simulink model "articulacion_q1"  (R2017b)
settings: Solver=VariableStepAuto  StartTime=0.0  StopTime=tmax  RelTol=1e-3
undefined symbols (not defined in the file): Beq, F_load_q1, f_pwm, Im_max, Jeq, Kdp, Kdv, Kip, Kiv, Km, Kpp, Kpv, Kt_q1, Kv_q1, Lm, Rm, ts, Vin_pwm, Vout_pwm
libraries: simulink x4
settings Model: Creator=JesusC  LastModifiedBy=JesusC

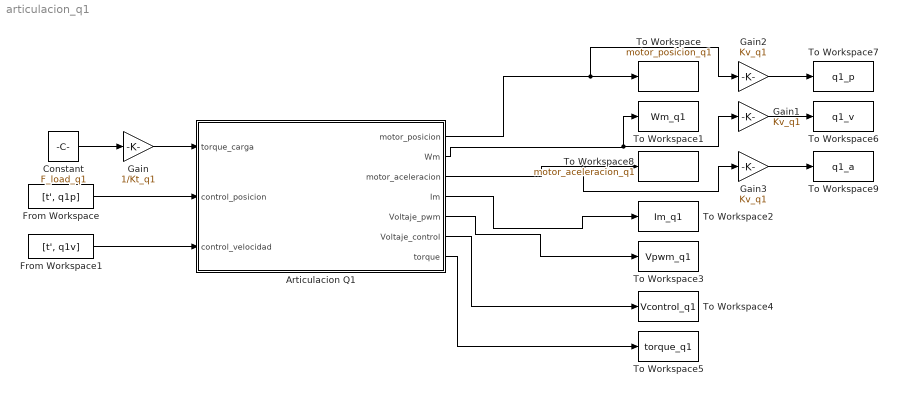
== system articulacion_q1 ==
  Articulacion Q1 : Subsystem
  Constant : Constant  Value=F_load_q1  VectorParams1D=off  SampleTime=ts
  From Workspace : FromWorkspace  VariableName=[t', q1p]  SampleTime=ts
  From Workspace1 : FromWorkspace  VariableName=[t', q1v]  SampleTime=ts
  Gain : Gain  Gain=1/Kt_q1
  Gain1 : Gain  Gain=Kv_q1
  Gain2 : Gain  Gain=Kv_q1
  Gain3 : Gain  Gain=Kv_q1
  To Workspace : ToWorkspace  VariableName=motor_posicion_q1  SampleTime=ts
      settings: MaxDataPoints=N
  To Workspace1 : ToWorkspace  VariableName=Wm_q1  SampleTime=ts
      settings: MaxDataPoints=N
  To Workspace2 : ToWorkspace  VariableName=Im_q1  SampleTime=ts
      settings: MaxDataPoints=N
  To Workspace3 : ToWorkspace  VariableName=Vpwm_q1  SampleTime=ts
      settings: MaxDataPoints=N
  To Workspace4 : ToWorkspace  VariableName=Vcontrol_q1  SampleTime=ts
      settings: MaxDataPoints=N
  To Workspace5 : ToWorkspace  VariableName=torque_q1  SampleTime=ts
      settings: MaxDataPoints=N
  To Workspace6 : ToWorkspace  VariableName=q1_v  SampleTime=ts
      settings: MaxDataPoints=N
  To Workspace7 : ToWorkspace  VariableName=q1_p  SampleTime=ts
      settings: MaxDataPoints=N
  To Workspace8 : ToWorkspace  VariableName=motor_aceleracion_q1  SampleTime=ts
      settings: MaxDataPoints=N
  To Workspace9 : ToWorkspace  VariableName=q1_a  SampleTime=ts
      settings: MaxDataPoints=N
  wires:
  Constant/1 -> Gain/1
  Gain1/1 -> To Workspace6/1
  Gain2/1 -> To Workspace7/1
  Articulacion Q1/6(Voltaje_control) -> To Workspace4/1
  Articulacion Q1/7(torque) -> To Workspace5/1
  Articulacion Q1/5(Voltaje_pwm) -> To Workspace3/1
  Articulacion Q1/4(Im) -> To Workspace2/1
  Articulacion Q1/2(Wm) -> Gain1/1, To Workspace1/1
  Articulacion Q1/1(motor_posicion) -> Gain2/1, To Workspace/1
  Articulacion Q1/3(motor_aceleracion) -> Gain3/1, To Workspace8/1
  Gain3/1 -> To Workspace9/1
  Gain/1 -> Articulacion Q1/1(torque_carga)
  From Workspace/1 -> Articulacion Q1/2(control_posicion)
  From Workspace1/1 -> Articulacion Q1/3(control_velocidad)

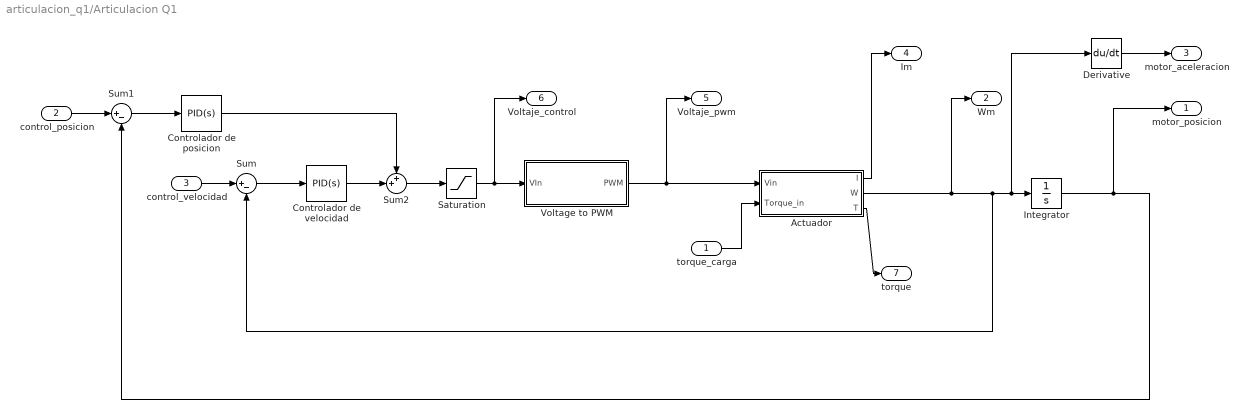
== system articulacion_q1/Articulacion Q1 ==
  torque_carga : Inport
  control_posicion : Inport  Port=2
  control_velocidad : Inport  Port=3
  "Actuador " : Subsystem
  Controlador de posicion : simulink/Continuous/PID Controller  Controller=PID  TimeDomain=Continuous-time  SampleTime=-1  IntegratorMethod=Forward Euler  FilterMethod=Forward Euler  Form=Parallel  UseFilter=on  ControllerParametersSource=internal  P=Kpp  I=Kip  D=Kdp  N=10000  InitialConditionSource=internal  InitialConditionForIntegrator=0  InitialConditionForFilter=0  ExternalReset=none  LimitOutput=off  UpperSaturationLimit=inf  LowerSaturationLimit=-inf  LinearizeAsGain=on  AntiWindupMode=none  Kb=1  TrackingMode=off  Kt=1  PParamMin=[]  PParamMax=[]  IParamMin=[]  IParamMax=[]  DParamMin=[]  DParamMax=[]  NParamMin=[]  NParamMax=[]  KbParamMin=[]  KbParamMax=[]  KtParamMin=[]  KtParamMax=[]  POutMin=[]  POutMax=[]  IOutMin=[]  IOutMax=[]  DOutMin=[]  DOutMax=[]  NOutMin=[]  NOutMax=[]  KbOutMin=[]  KbOutMax=[]  KtOutMin=[]  KtOutMax=[]  IntegratorOutMin=[]  IntegratorOutMax=[]  FilterOutMin=[]  FilterOutMax=[]  SumOutMin=[]  SumOutMax=[]  SumI1OutMin=[]  SumI1OutMax=[]  SumI2OutMin=[]  SumI2OutMax=[]  SumI3OutMin=[]  SumI3OutMax=[]  SumDOutMin=[]  SumDOutMax=[]  SaturationOutMin=[]  SaturationOutMax=[]  IntegratorContinuousStateAttributes=''  IntegratorStateMustResolveToSignalObject=off  IntegratorRTWStateStorageClass=Auto  FilterContinuousStateAttributes=''  FilterStateMustResolveToSignalObject=off  FilterRTWStateStorageClass=Auto  DifferentiatorICPrevScaledInput=0  DifferentiatorOutMin=[]  DifferentiatorOutMax=[]  InitialConditionSetting=State (most efficient)  FilterDiffOutCoefMin=[]  FilterDiffOutCoefMax=[]  SumDenOutMin=[]  SumDenOutMax=[]  SumNumOutMin=[]  SumNumOutMax=[]  ReciprocalOutMin=[]  ReciprocalOutMax=[]  DivideOutMin=[]  DivideOutMax=[]  TunerSelectOption=Transfer Function Based (PID Tuner App)
  Controlador de velocidad : simulink/Continuous/PID Controller  Controller=PID  TimeDomain=Continuous-time  SampleTime=-1  IntegratorMethod=Forward Euler  FilterMethod=Forward Euler  Form=Parallel  UseFilter=on  ControllerParametersSource=internal  P=Kpv  I=Kiv  D=Kdv  N=10000  InitialConditionSource=internal  InitialConditionForIntegrator=0  InitialConditionForFilter=0  ExternalReset=none  LimitOutput=off  UpperSaturationLimit=inf  LowerSaturationLimit=-inf  LinearizeAsGain=on  AntiWindupMode=none  Kb=1  TrackingMode=off  Kt=1  PParamMin=[]  PParamMax=[]  IParamMin=[]  IParamMax=[]  DParamMin=[]  DParamMax=[]  NParamMin=[]  NParamMax=[]  KbParamMin=[]  KbParamMax=[]  KtParamMin=[]  KtParamMax=[]  POutMin=[]  POutMax=[]  IOutMin=[]  IOutMax=[]  DOutMin=[]  DOutMax=[]  NOutMin=[]  NOutMax=[]  KbOutMin=[]  KbOutMax=[]  KtOutMin=[]  KtOutMax=[]  IntegratorOutMin=[]  IntegratorOutMax=[]  FilterOutMin=[]  FilterOutMax=[]  SumOutMin=[]  SumOutMax=[]  SumI1OutMin=[]  SumI1OutMax=[]  SumI2OutMin=[]  SumI2OutMax=[]  SumI3OutMin=[]  SumI3OutMax=[]  SumDOutMin=[]  SumDOutMax=[]  SaturationOutMin=[]  SaturationOutMax=[]  IntegratorContinuousStateAttributes=''  IntegratorStateMustResolveToSignalObject=off  IntegratorRTWStateStorageClass=Auto  FilterContinuousStateAttributes=''  FilterStateMustResolveToSignalObject=off  FilterRTWStateStorageClass=Auto  DifferentiatorICPrevScaledInput=0  DifferentiatorOutMin=[]  DifferentiatorOutMax=[]  InitialConditionSetting=State (most efficient)  FilterDiffOutCoefMin=[]  FilterDiffOutCoefMax=[]  SumDenOutMin=[]  SumDenOutMax=[]  SumNumOutMin=[]  SumNumOutMax=[]  ReciprocalOutMin=[]  ReciprocalOutMax=[]  DivideOutMin=[]  DivideOutMax=[]  TunerSelectOption=Transfer Function Based (PID Tuner App)
  Derivative : Derivative  CoefficientInTFapproximation=0
  Integrator : Integrator
  Saturation : Saturate  UpperLimit=Vin_pwm  LowerLimit=-Vin_pwm
  Sum : Sum  Inputs=|+-
  Sum1 : Sum  Inputs=|+-
  Sum2 : Sum  Inputs=++|
  Voltage to PWM : Subsystem
  motor_posicion : Outport
  Wm : Outport  Port=2
  motor_aceleracion : Outport  Port=3
  Im : Outport  Port=4
  Voltaje_pwm : Outport  Port=5
  Voltaje_control : Outport  Port=6
  torque : Outport  Port=7
  wires:
  Derivative/1 -> motor_aceleracion/1
  Integrator/1 -> motor_posicion/1, Sum1/2
  control_posicion/1 -> Sum1/1
  "Actuador "/1(I) -> Im/1
  "Actuador "/3(T) -> torque/1
  Sum2/1 -> Saturation/1
  Sum1/1 -> Controlador de posicion/1
  torque_carga/1 -> "Actuador "/2(Torque_in)
  Voltage to PWM/1(PWM) -> Voltaje_pwm/1, "Actuador "/1(Vin)
  Saturation/1 -> Voltaje_control/1, Voltage to PWM/1(VIn)
  control_velocidad/1 -> Sum/1
  "Actuador "/2(W) -> Wm/1, Sum/2, Derivative/1, Integrator/1
  Sum/1 -> Controlador de velocidad/1
  Controlador de velocidad/1 -> Sum2/2
  Controlador de posicion/1 -> Sum2/1

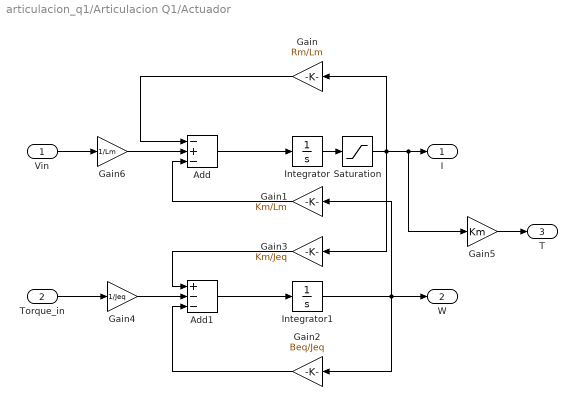
== system articulacion_q1/Articulacion Q1/Actuador  ==
  Vin : Inport
  Torque_in : Inport  Port=2
  Add : Sum  Inputs=-+-
  Add1 : Sum  Inputs=+--
  Gain : Gain  Gain=Rm/Lm
  Gain1 : Gain  Gain=Km/Lm
  Gain2 : Gain  Gain=Beq/Jeq
  Gain3 : Gain  Gain=Km/Jeq
  Gain4 : Gain  Gain=1/Jeq
  Gain5 : Gain  Gain=Km
  Gain6 : Gain  Gain=1/Lm
  Integrator : Integrator
  Integrator1 : Integrator
  Saturation : Saturate  UpperLimit=Im_max  LowerLimit=-Im_max
  I : Outport
  W : Outport  Port=2
  T : Outport  Port=3
  wires:
  Integrator/1 -> Saturation/1
  Gain/1 -> Add/1
  Integrator1/1 -> Gain2/1, Gain1/1, W/1
  Gain1/1 -> Add/3
  Add/1 -> Integrator/1
  Add1/1 -> Integrator1/1
  Gain2/1 -> Add1/3
  Gain3/1 -> Add1/1
  Torque_in/1 -> Gain4/1
  Gain4/1 -> Add1/2
  Gain5/1 -> T/1
  Vin/1 -> Gain6/1
  Gain6/1 -> Add/2
  Saturation/1 -> Gain3/1, Gain/1, Gain5/1, I/1

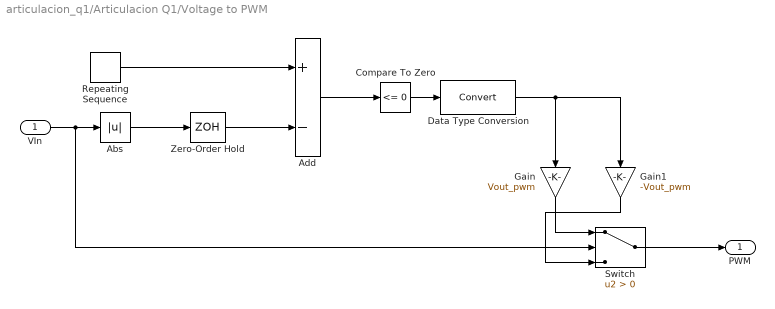
== system articulacion_q1/Articulacion Q1/Voltage to PWM ==
  VIn : Inport
  Abs : Abs
  Add : Sum  Inputs=+-
  Compare To Zero : simulink/Logic and Bit Operations/Compare To Zero  relop=<=  OutDataTypeStr=boolean
  Data Type Conversion : DataTypeConversion
  Gain : Gain  Gain=Vout_pwm
  Gain1 : Gain  Gain=-Vout_pwm
  Repeating Sequence : simulink/Sources/Repeating Sequence  rep_seq_t=[0 1/f_pwm]  rep_seq_y=[0 Vin_pwm]
  Switch : Switch  Criteria=u2 > Threshold
  Zero-Order Hold : ZeroOrderHold  SampleTime=-1
  PWM : Outport
  wires:
  Repeating Sequence/1 -> Add/1
  Add/1 -> Compare To Zero/1
  Zero-Order Hold/1 -> Add/2
  Abs/1 -> Zero-Order Hold/1
  VIn/1 -> Switch/2, Abs/1
  Gain/1 -> Switch/1
  Gain1/1 -> Switch/3
  Compare To Zero/1 -> Data Type Conversion/1
  Switch/1 -> PWM/1
  Data Type Conversion/1 -> Gain/1, Gain1/1
